simulink model "sim_closedloop_position_controller_2022b"  (R2022b)
settings: Solver=FixedStepAuto  StartTime=0.0  StopTime=10.0  FixedStep=0.05  RelTol=1e-3
undefined symbols (not defined in the file or in its folder): A, B, Ki, Kp
settings Model: Creator=RAOUF  LastModifiedBy=Claudia Yasar
settings DataIOCC: ReturnWorkspaceOutputs=off
settings OptimizationCC: ReuseModelBlockBuffer=on

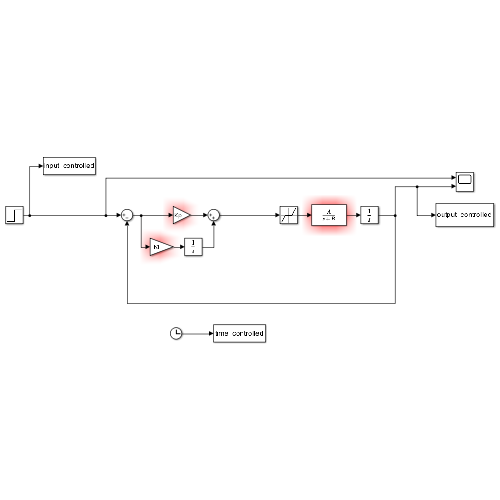
[thumbnail: Simulink's stored preview of the top-level diagram]
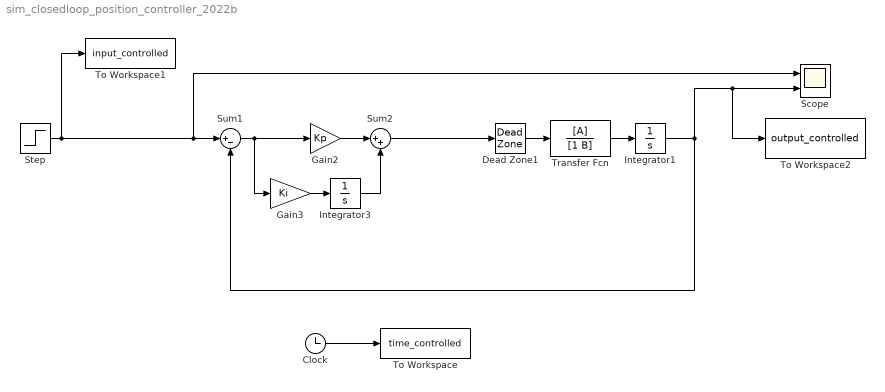
== system sim_closedloop_position_controller_2022b ==
  Clock : Clock
  Dead Zone1 : DeadZone  LowerValue=-0.05  UpperValue=0.05
  Gain2 : Gain  Gain=Kp
  Gain3 : Gain  Gain=Ki
  Integrator1 : Integrator
  Integrator3 : Integrator
  Scope : Scope  NumInputPorts=2
  Step : Step  After=pi/2  SampleTime=0
  Sum1 : Sum  Inputs=|+-
  Sum2 : Sum  Inputs=|++
  To Workspace : ToWorkspace  VariableName=time_controlled  SampleTime=-1
      settings: Save2DSignal=2-D array (concatenate along first dimension)
  To Workspace1 : ToWorkspace  VariableName=input_controlled  SampleTime=-1
      settings: Save2DSignal=2-D array (concatenate along first dimension)
  To Workspace2 : ToWorkspace  VariableName=output_controlled  SampleTime=-1
      settings: Save2DSignal=2-D array (concatenate along first dimension)
  Transfer Fcn : TransferFcn  Numerator=[A]  Denominator=[1 B]
  wires:
  Sum2/1 -> Dead Zone1/1
  Integrator3/1 -> Sum2/2
  Gain2/1 -> Sum2/1
  Transfer Fcn/1 -> Integrator1/1
  Integrator1/1 -> To Workspace2/1, Scope/2, Sum1/2
  Sum1/1 -> Gain3/1, Gain2/1
  Gain3/1 -> Integrator3/1
  Step/1 -> To Workspace1/1, Scope/1, Sum1/1
  Dead Zone1/1 -> Transfer Fcn/1
  Clock/1 -> To Workspace/1
